simulink model "compare_height"  (R2018b)
settings: Solver=VariableStepAuto  StartTime=0.0  StopTime=50.0  MaxStep=0.02  RelTol=1e-3
libraries: simulink x2
settings Model: Creator=73508  LastModifiedBy=73508

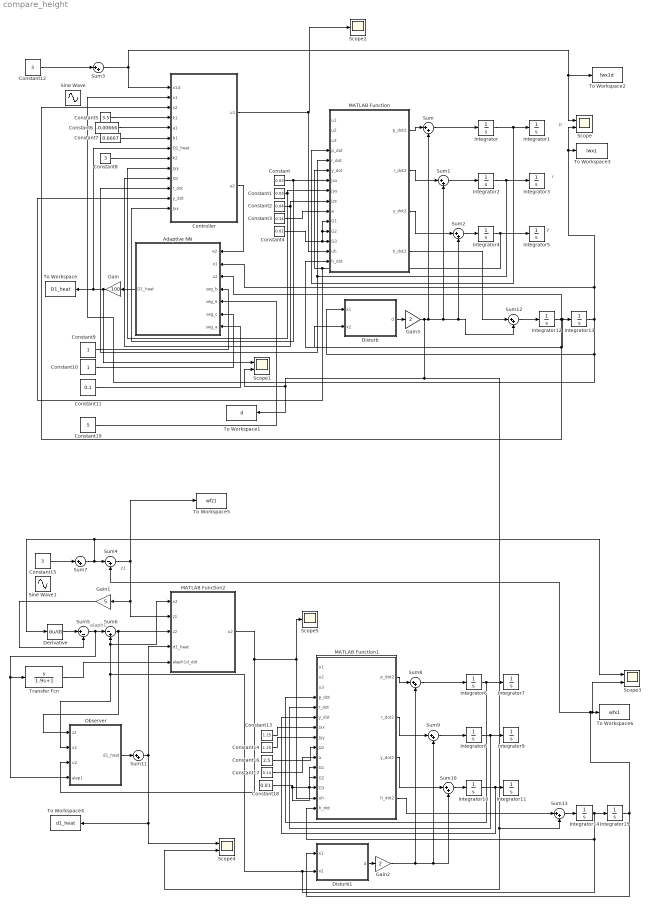
== system compare_height ==
  note: r
  note: y
  note: p
  note: alaph1
  note: z1
  Adaptive NN : Subsystem
  Constant : Constant  Value=0.03
  Constant1 : Constant  Value=0.03
  Constant10 : Constant
  Constant11 : Constant  Value=0.1
  Constant12 : Constant  Value=3
  Constant13 : Constant  Value=1.25
  Constant14 : Constant  Value=1.25
  Constant15 : Constant  Value=3
  Constant16 : Constant  Value=2.5
  Constant17 : Constant  Value=0.14
  Constant18 : Constant  Value=0.01
  Constant19 : Constant  Value=5
  Constant2 : Constant  Value=0.04
  Constant3 : Constant  Value=0.14
  Constant4 : Constant  Value=0.01
  Constant5 : Constant  Value=3.5
  Constant6 : Constant  Value=-0.00666
  Constant7 : Constant  Value=0.6667
  Constant8 : Constant  Value=3
  Constant9 : Constant
  Controller : Subsystem
  Derivative : Derivative
  Disturb : Subsystem
  Disturb1 : Subsystem
  Gain : Gain  Gain=100
  Gain1 : Gain  Gain=5
  Gain2 : Gain  Gain=2
  Gain3 : Gain  Gain=2
  Integrator{,1..15} (16 alike) : Integrator
  MATLAB Function : MATLAB Function  TreatAsAtomicUnit=on
  MATLAB Function1 : MATLAB Function  TreatAsAtomicUnit=on
  MATLAB Function2 : MATLAB Function  TreatAsAtomicUnit=on
  Observer : Subsystem
  Scope{,1,3..4} (4 alike) : Scope  NumInputPorts=2
  Scope2 : Scope
  Scope5 : Scope
  Sine Wave : Sin  Amplitude=0.5  Frequency=0.08*pi  Phase=0.5*pi  SampleTime=0
  Sine Wave1 : Sin  Amplitude=0.5  Frequency=0.08*pi  Phase=0.5*pi  SampleTime=0
  Sum{,1..3,7..13} (11 alike) : Sum  Inputs=|++
  Sum4 : Sum  Inputs=|-+
  Sum5 : Sum  Inputs=|+-
  Sum6 : Sum  Inputs=|-+
  To Workspace : ToWorkspace  VariableName=D1_heat  SampleTime=-1
  To Workspace1 : ToWorkspace  VariableName=d  SampleTime=-1
  To Workspace2 : ToWorkspace  VariableName=lwx1d  SampleTime=-1
  To Workspace3 : ToWorkspace  VariableName=lwx1  SampleTime=-1
  To Workspace4 : ToWorkspace  VariableName=d1_heat  SampleTime=-1
  To Workspace5 : ToWorkspace  VariableName=wfz1  SampleTime=-1
  To Workspace6 : ToWorkspace  VariableName=wfx1  SampleTime=-1
  Transfer Fcn : TransferFcn  Numerator=[1 0]  Denominator=[1.9 1]
  wires:
  Sum2/1 -> Integrator4/1
  Adaptive NN/1(D1_heat) -> Gain/1
  Integrator/1 -> MATLAB Function/4(p_dot), Integrator1/1
  Integrator4/1 -> MATLAB Function/6(y_dot), Controller/12(y_dot), Integrator5/1
  Sum3/1 -> Controller/1(x1d), To Workspace2/1, Scope/1
  MATLAB Function/1(p_dot2) -> Sum/1
  Constant5/1 -> Controller/4(k1)
  Constant6/1 -> Controller/5(a1)
  Constant4/1 -> MATLAB Function/13(G3), MATLAB Function/12(G2), MATLAB Function/11(G1)
  Constant9/1 -> Adaptive NN/4(seg_b)
  Constant10/1 -> Adaptive NN/6(seg_c)
  Controller/2(e2) -> Adaptive NN/1(e2)
  Constant7/1 -> Controller/6(b1)
  MATLAB Function/2(r_dot2) -> Sum1/1
  Gain3/1 -> Scope4/2, Sum13/2, Scope1/2, To Workspace1/1, Sum/2, Sum1/2, Sum12/2, Sum2/2
  MATLAB Function/3(y_dot2) -> Sum2/1
  Sum1/1 -> Integrator2/1
  Controller/1(u1) -> Scope2/1, MATLAB Function/14(uh)
  Constant/1 -> Controller/13(Jxx), MATLAB Function/7(Jxx)
  Sum/1 -> Integrator/1
  Constant11/1 -> Adaptive NN/7(seg_a)
  Gain/1 -> Scope1/1, To Workspace/1, Controller/7(D1_heat)
  Integrator2/1 -> MATLAB Function/5(r_dot), Controller/11(r_dot), Integrator3/1
  Constant2/1 -> Controller/10(Jzz), MATLAB Function/9(Jzz)
  Constant3/1 -> MATLAB Function/10(a)
  Constant8/1 -> Controller/8(k2)
  Constant1/1 -> Controller/9(Jyy), MATLAB Function/8(Jyy)
  Sum10/1 -> Integrator10/1
  Gain2/1 -> Sum9/2, Sum10/2, Sum8/2
  Transfer Fcn/1 -> MATLAB Function2/5(alaph1d_dot)
  Derivative/1 -> Sum5/1
  Sum5/1 -> Transfer Fcn/1, Observer/4(alap1), Sum6/1
  Sum6/1 -> Observer/1(z2), MATLAB Function2/3(z2)
  Constant17/1 -> MATLAB Function1/10(a)
  MATLAB Function1/2(r_dot2) -> Sum9/1
  Constant14/1 -> MATLAB Function1/8(Jyy)
  Gain1/1 -> Sum5/2
  Sum11/1 -> To Workspace4/1, Scope4/1, MATLAB Function2/4(d1_heat)
  Constant18/1 -> MATLAB Function1/13(G3), MATLAB Function1/11(G1), MATLAB Function1/12(G2)
  MATLAB Function1/1(p_dot2) -> Sum8/1
  Sum4/1 -> To Workspace5/1, MATLAB Function2/2(z1), Gain1/1
  Sum8/1 -> Integrator6/1
  Integrator10/1 -> MATLAB Function1/6(y_dot), Integrator11/1
  Sum9/1 -> Integrator8/1
  Integrator6/1 -> MATLAB Function1/4(p_dot), Integrator7/1
  Integrator8/1 -> MATLAB Function1/5(r_dot), Integrator9/1
  MATLAB Function1/3(y_dot2) -> Sum10/1
  Constant13/1 -> MATLAB Function1/7(Jxx)
  Constant16/1 -> MATLAB Function1/9(Jzz)
  Observer/1(d1_heat) -> Sum11/1
  Sum7/1 -> Derivative/1, Scope3/1, Sum4/1
  MATLAB Function2/1(u2) -> MATLAB Function1/14(uh), Scope5/1, Observer/3(u2)
  Constant19/1 -> Adaptive NN/5(seg_e)
  Disturb1/1(d) -> Gain2/1
  Disturb/1(d) -> Gain3/1
  Constant15/1 -> Sum7/1
  Constant12/1 -> Sum3/1
  Integrator12/1 -> Disturb/2(x2), Controller/3(x2), Adaptive NN/3(x2), MATLAB Function/15(h_dot), Integrator13/1
  Sum12/1 -> Integrator12/1
  MATLAB Function/4(h_dot2) -> Sum12/1
  Integrator13/1 -> Scope/2, To Workspace3/1, Adaptive NN/2(x1), Disturb/1(x1), Controller/2(x1)
  MATLAB Function1/4(h_dot2) -> Sum13/1
  Sum13/1 -> Integrator14/1
  Integrator14/1 -> MATLAB Function2/1(x2), Sum6/2, Observer/2(x2), Disturb1/2(x2), MATLAB Function1/15(h_dot), Integrator15/1
  Integrator15/1 -> Sum4/2, Scope3/2, To Workspace6/1, Disturb1/1(x1)

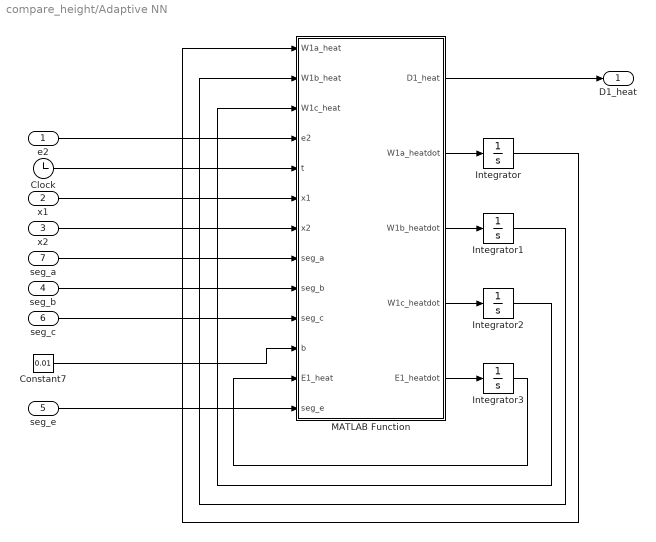
== system compare_height/Adaptive NN ==
  e2 : Inport
  x1 : Inport  Port=2
  x2 : Inport  Port=3
  seg_b : Inport  Port=4
  seg_e : Inport  Port=5
  seg_c : Inport  Port=6
  seg_a : Inport  Port=7
  Clock : Clock
  Constant7 : Constant  Value=0.01
  Integrator{,1..3} (4 alike) : Integrator
  MATLAB Function : MATLAB Function  InitFcn=|  TreatAsAtomicUnit=on
      | W1b_heat = zeros(21,1);
      | W1c_heat = zeros(15,1);
      | W1a_heat = zeros(315,1);
      | W1b_heatdot = zeros(21,1);
      | W1c_heatdot = zeros(15,1);
      | W1a_heatdot = zeros(315,1);
  D1_heat : Outport
  wires:
  e2/1 -> MATLAB Function/4(e2)
  MATLAB Function/1(D1_heat) -> D1_heat/1
  MATLAB Function/4(W1c_heatdot) -> Integrator2/1
  MATLAB Function/3(W1b_heatdot) -> Integrator1/1
  MATLAB Function/2(W1a_heatdot) -> Integrator/1
  Integrator/1 -> MATLAB Function/1(W1a_heat)
  Integrator1/1 -> MATLAB Function/2(W1b_heat)
  Integrator2/1 -> MATLAB Function/3(W1c_heat)
  Clock/1 -> MATLAB Function/5(t)
  x1/1 -> MATLAB Function/6(x1)
  x2/1 -> MATLAB Function/7(x2)
  seg_b/1 -> MATLAB Function/9(seg_b)
  seg_c/1 -> MATLAB Function/10(seg_c)
  seg_a/1 -> MATLAB Function/8(seg_a)
  MATLAB Function/5(E1_heatdot) -> Integrator3/1
  Integrator3/1 -> MATLAB Function/12(E1_heat)
  Constant7/1 -> MATLAB Function/11(b)
  seg_e/1 -> MATLAB Function/13(seg_e)

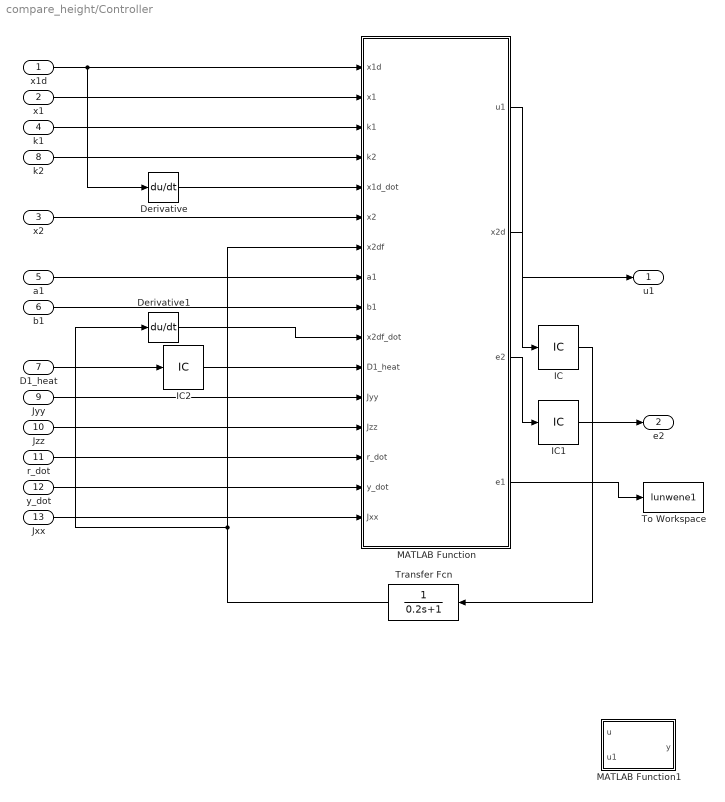
== system compare_height/Controller ==
  x1d : Inport
  x1 : Inport  Port=2
  x2 : Inport  Port=3
  k1 : Inport  Port=4
  a1 : Inport  Port=5
  b1 : Inport  Port=6
  D1_heat : Inport  Port=7
  k2 : Inport  Port=8
  Jyy : Inport  Port=9
  Jzz : Inport  Port=10
  r_dot : Inport  Port=11
  y_dot : Inport  Port=12
  Jxx : Inport  Port=13
  Derivative : Derivative
  Derivative1 : Derivative
  IC : InitialCondition  Value=0
  IC1 : InitialCondition  Value=0
  IC2 : InitialCondition  Value=0
  MATLAB Function : MATLAB Function  TreatAsAtomicUnit=on
  MATLAB Function1 : MATLAB Function  TreatAsAtomicUnit=on
  To Workspace : ToWorkspace  VariableName=lunwene1  SampleTime=-1
  Transfer Fcn : TransferFcn  Denominator=[0.2 1]
  u1 : Outport
  e2 : Outport  Port=2
  wires:
  x1d/1 -> Derivative/1, MATLAB Function/1(x1d)
  x1/1 -> MATLAB Function/2(x1)
  x2/1 -> MATLAB Function/6(x2)
  k1/1 -> MATLAB Function/3(k1)
  a1/1 -> MATLAB Function/8(a1)
  b1/1 -> MATLAB Function/9(b1)
  MATLAB Function/1(u1) -> u1/1
  MATLAB Function/2(x2d) -> IC/1
  MATLAB Function/3(e2) -> IC1/1
  Derivative/1 -> MATLAB Function/5(x1d_dot)
  Derivative1/1 -> MATLAB Function/10(x2df_dot)
  D1_heat/1 -> IC2/1
  k2/1 -> MATLAB Function/4(k2)
  Transfer Fcn/1 -> MATLAB Function/7(x2df), Derivative1/1
  IC/1 -> Transfer Fcn/1
  IC1/1 -> e2/1
  IC2/1 -> MATLAB Function/11(D1_heat)
  MATLAB Function/4(e1) -> To Workspace/1
  Jyy/1 -> MATLAB Function/12(Jyy)
  Jzz/1 -> MATLAB Function/13(Jzz)
  r_dot/1 -> MATLAB Function/14(r_dot)
  Jxx/1 -> MATLAB Function/16(Jxx)
  y_dot/1 -> MATLAB Function/15(y_dot)

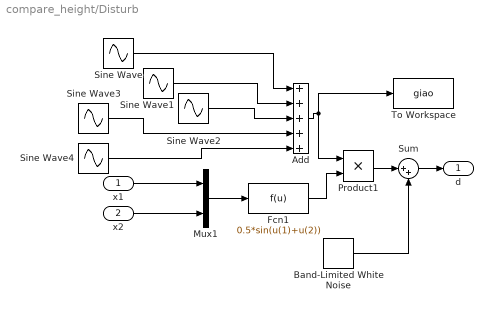
== system compare_height/Disturb ==
  x1 : Inport
  x2 : Inport  Port=2
  Add : Sum  Inputs=+++++
  Band-Limited White Noise : simulink/Sources/Band-Limited White Noise  Cov=[0.00001]  Ts=0.01  seed=[23341]
  Fcn1 : Fcn  Expr=0.5*sin(u(1)+u(2))
  Mux1 : Mux  Inputs=2
  Product1 : Product
  Sine Wave : Sin  SampleTime=0
  Sine Wave1 : Sin  Amplitude=0.39  Frequency=2.56  SampleTime=0
  Sine Wave2 : Sin  Amplitude=0.2  Frequency=5  SampleTime=0
  Sine Wave3 : Sin  Amplitude=0.14  Frequency=7  SampleTime=0
  Sine Wave4 : Sin  Amplitude=0.33  Frequency=3  SampleTime=0
  Sum : Sum  Inputs=|++
  To Workspace : ToWorkspace  VariableName=giao  SampleTime=-1
  d : Outport
  wires:
  x2/1 -> Mux1/2
  Sine Wave2/1 -> Add/3
  Sine Wave/1 -> Add/1
  Sine Wave1/1 -> Add/2
  Fcn1/1 -> Product1/2
  x1/1 -> Mux1/1
  Sine Wave3/1 -> Add/4
  Mux1/1 -> Fcn1/1
  Add/1 -> To Workspace/1, Product1/1
  Product1/1 -> Sum/1
  Sum/1 -> d/1
  Band-Limited White Noise/1 -> Sum/2
  Sine Wave4/1 -> Add/5

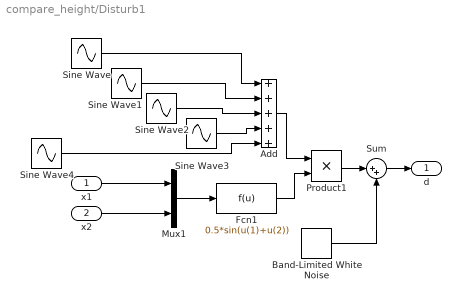
== system compare_height/Disturb1 ==
  x1 : Inport
  x2 : Inport  Port=2
  Add : Sum  Inputs=+++++
  Band-Limited White Noise : simulink/Sources/Band-Limited White Noise  Cov=[0.00001]  Ts=0.011  seed=[23341]
  Fcn1 : Fcn  Expr=0.5*sin(u(1)+u(2))
  Mux1 : Mux  Inputs=2
  Product1 : Product
  Sine Wave : Sin  SampleTime=0
  Sine Wave1 : Sin  Amplitude=0.33  Frequency=3  SampleTime=0
  Sine Wave2 : Sin  Amplitude=0.2  Frequency=5  SampleTime=0
  Sine Wave3 : Sin  Amplitude=0.14  Frequency=7  SampleTime=0
  Sine Wave4 : Sin  Amplitude=0.33  Frequency=3  SampleTime=0
  Sum : Sum  Inputs=|++
  d : Outport
  wires:
  x2/1 -> Mux1/2
  Sine Wave2/1 -> Add/3
  Sine Wave/1 -> Add/1
  Sine Wave1/1 -> Add/2
  Fcn1/1 -> Product1/2
  x1/1 -> Mux1/1
  Sine Wave3/1 -> Add/4
  Mux1/1 -> Fcn1/1
  Add/1 -> Product1/1
  Product1/1 -> Sum/1
  Sum/1 -> d/1
  Band-Limited White Noise/1 -> Sum/2
  Sine Wave4/1 -> Add/5

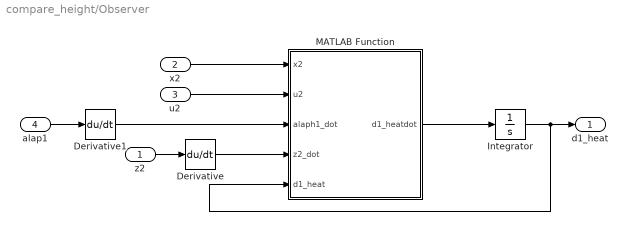
== system compare_height/Observer ==
  z2 : Inport
  x2 : Inport  Port=2
  u2 : Inport  Port=3
  alap1 : Inport  Port=4
  Derivative : Derivative
  Derivative1 : Derivative
  Integrator : Integrator
  MATLAB Function : MATLAB Function  TreatAsAtomicUnit=on
  d1_heat : Outport
  wires:
  MATLAB Function/1(d1_heatdot) -> Integrator/1
  u2/1 -> MATLAB Function/2(u2)
  x2/1 -> MATLAB Function/1(x2)
  z2/1 -> Derivative/1
  Derivative/1 -> MATLAB Function/4(z2_dot)
  Integrator/1 -> MATLAB Function/5(d1_heat), d1_heat/1
  alap1/1 -> Derivative1/1
  Derivative1/1 -> MATLAB Function/3(alaph1_dot)

== matlab function compare_height/Controller/MATLAB Function ==
  data: x1d input; u1 output; x1 input; k1 input; k2 input; x1d_dot input; x2 input; x2df input; a1 input; b1 input; x2df_dot input; D1_heat input; x2d output; e2 output; e1 output; Jyy input; Jzz input; r_dot input; y_dot input; Jxx input
function [u1,x2d,e2,e1] = controller(x1d,x1,k1,k2,x1d_dot,x2,x2df,a1,b1,x2df_dot,D1_heat,Jyy,Jzz,r_dot,y_dot,Jxx)
    e1 = x1-x1d;
    x2d = -k1*e1+x1d_dot;
    e2 = x2-x2df;
    c1=-9.8;
    u1 = (-k2*e2-a1*x2-D1_heat+x2df_dot-c1)/b1;
end

== matlab function compare_height/MATLAB Function ==
  data: u1 input; p_dot2 output; u2 input; u3 input; p_dot input; r_dot input; y_dot input; Jxx input; Jyy input; Jzz input; a input; G1 input; G2 input; G3 input; r_dot2 output; y_dot2 output; uh input; h_dot input; h_dot2 output
function [p_dot2,r_dot2,y_dot2,h_dot2] = Attitude_dynamics(u1,u2,u3,p_dot,r_dot,y_dot,Jxx,Jyy,Jzz,a,G1,G2,G3,uh,h_dot)
    p_dot2 = a*u1/Jxx-G1*a*p_dot/Jxx+(Jyy-Jzz)*r_dot*y_dot/Jxx;
    r_dot2 = a*u2/Jzz-G2*a*r_dot/Jzz+(Jxx-Jyy)*p_dot*y_dot/Jzz;
    y_dot2 = a*u3/Jyy-G3*a*y_dot/Jyy+(Jxx-Jzz)*r_dot*p_dot/Jyy;
    h_dot2 = -G1/1.5*h_dot+uh/1.5-9.8;
end

== matlab function compare_height/Adaptive NN/MATLAB Function ==
  data: W1a_heat input size=[315,1]; D1_heat output; W1b_heat input size=[21,1]; W1c_heat input size=[15,1]; e2 input; W1a_heatdot output size=[315,1]; W1b_heatdot output size=[21,1]; W1c_heatdot output size=[15,1]; t input; x1 input; x2 input; seg_a input; seg_b input; seg_c input; b input; E1_heat input; seg_e input; E1_heatdot output
function [D1_heat,W1a_heatdot,W1b_heatdot,W1c_heatdot,E1_heatdot] = fcn(W1a_heat,W1b_heat,W1c_heat,e2,t,x1,x2,seg_a,seg_b,seg_c,b,E1_heat,seg_e)
%%%%%%%%%%%%%%%%%%%%%%神经网络b
    cbij=[-1 -0.9 -0.8 -0.7 -0.6 -0.5 -0.4 -0.3 -0.2 -0.1 0 0.1 0.2 0.3 0.4 0.5 0.6 0.7 0.8 0.9 1 ;
     -2 -1.8 -1.6 -1.4 -1.2 -1 -0.8 -0.6 -0.4 -0.2 0 0.2 0.4 0.6 0.8 1 1.2 1.4 1.6 1.8 2];%21
    bbj = [0.2;0.2;0.2;0.2;0.2;0.2;0.2;0.2;0.2;0.2;0.2;0.2;0.2;0.2;0.2;0.2;0.2;0.2;0.2;0.2;0.2];
    S_b=zeros(21,1);
    Jb = [x1;x2];
   for j=1:1:21
        S_b(j)=exp(-norm(Jb-cbij(:,j))^(2)/(2*bbj(j)^(2)));
   end
   dbd =W1b_heat'*S_b;
   W1b_heatdot = -seg_b*W1b_heat+S_b*e2;
   %%%%%%%%%%%%%%%%%%%%%%神经网络c
   S_c = zeros(15,1);
   for j =1:1:15
       S_c(j)=sin(j*t);
   end
   dcd = W1c_heat'*S_c;
   W1c_heatdot = -seg_c*W1c_heat+S_c*e2;
    %%%%%%%%%%%%%%%%%%%%%%神经网络a
    S_a = zeros(315,1);
    for i = 0:1:14
        for j = 1:1:21
            S_a(j+21*i) = exp(-norm(Jb-cbij(:,j))^(2)/(2*bbj(j)^(2)))*sin((i+1)*t);
        end
    end
    dad = W1a_heat'*S_a;
    W1a_heatdot = -seg_a*W1a_heat+S_a*e2;
    E1_heatdot = -seg_e*E1_heat+e2*tanh(e2/b);
    ded = E1_heatdot*tanh(e2/b);
   D1_heat = dad+dbd+dcd+ded;
end

== matlab function compare_height/Controller/MATLAB Function1 ==
  data: u input; y output; u1 input
function y = fcn(u,u1)

y = u;

== matlab function compare_height/MATLAB Function1 ==
  data: u1 input; p_dot2 output; u2 input; u3 input; p_dot input; r_dot input; y_dot input; Jxx input; Jyy input; Jzz input; a input; G1 input; G2 input; G3 input; r_dot2 output; y_dot2 output; uh input; h_dot input; h_dot2 output
function [p_dot2,r_dot2,y_dot2,h_dot2] = Attitude_dynamics(u1,u2,u3,p_dot,r_dot,y_dot,Jxx,Jyy,Jzz,a,G1,G2,G3,uh,h_dot)
   p_dot2 = a*u1/Jxx-G1*a*p_dot/Jxx+(Jyy-Jzz)*r_dot*y_dot/Jxx;
    r_dot2 = a*u2/Jzz-G2*a*r_dot/Jzz+(Jxx-Jyy)*p_dot*y_dot/Jzz;
    y_dot2 = a*u3/Jyy-G3*a*y_dot/Jyy+(Jxx-Jzz)*r_dot*p_dot/Jyy;
    h_dot2 = -G1/1.5*h_dot+uh/1.5-9.8;
end

== matlab function compare_height/MATLAB Function2 ==
  data: x2 input; u2 output [-20..20]; z1 input; z2 input; d1_heat input; alaph1d_dot input
function u2  = controller(x2,z1,z2,d1_heat,alaph1d_dot)
    a = 0.2;jxx=1.25;jyy=1.25;jzz=2.5;G4 =0.012; G5 =0.012; G6 =0.012;c2 = 5;kb1 =0.0005;
    a1 = -0.00666;
    b1 = 0.6667;
    u2 = (-a1*x2-c2*z2-d1_heat+alaph1d_dot-(z1/(kb1^2-z1^2)))/b1;
end

== matlab function compare_height/Observer/MATLAB Function ==
  data: x2 input; d1_heatdot output size=1; u2 input; alaph1_dot input; z2_dot input; d1_heat input
function d1_heatdot = fcn(x2,u2,alaph1_dot,z2_dot,d1_heat)
     a = 0.2;jxx=1.25;jyy=1.25;jzz=2.5;G4 =0.012; G5 =0.012; G6 =0.012;c2 = 5;kb1 =0.0005;l1 = 1.005;
      a1 = -0.00666;
         b1 =0.6667;
     p1_dot = -l1*(a1*x2+b1*u2+d1_heat-alaph1_dot);
     d1_heatdot = p1_dot+l1*z2_dot;
 
end
